simulink model "model"  (R2020a)
settings: Solver=VariableStepAuto  StartTime=0.0  StopTime=10  RelTol=1e-3
undefined symbols (not defined in the file): b, F, k1, k2, m1, m2
settings Model: Creator=PRATIKSHA  LastModifiedBy=PRATIKSHA

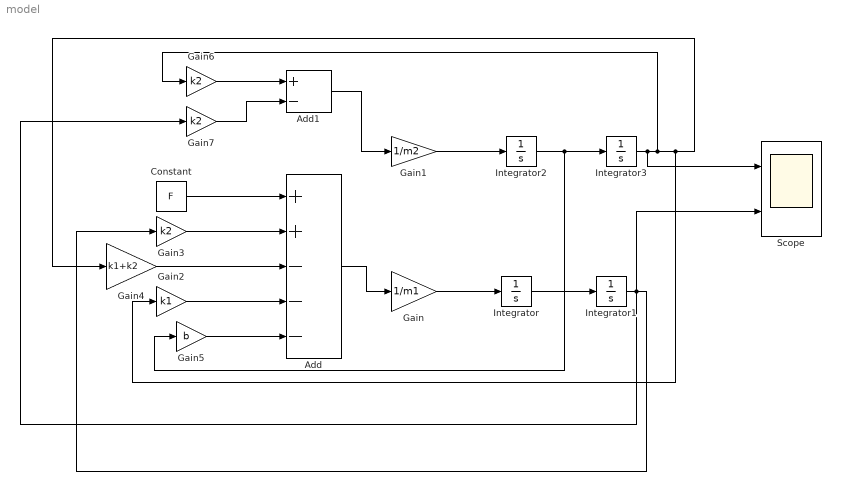
== system model ==
  Add : Sum  Inputs=++---
  Add1 : Sum  Inputs=+-
  Constant : Constant  Value=F
  Gain : Gain  Gain=1/m1
  Gain1 : Gain  Gain=1/m2
  Gain2 : Gain  Gain=k1
  Gain3 : Gain  Gain=k2
  Gain4 : Gain  Gain=k1+k2
  Gain5 : Gain  Gain=b
  Gain6 : Gain  Gain=k2
  Gain7 : Gain  Gain=k2
  Integrator{,1..3} (4 alike) : Integrator
  Scope : Scope  NumInputPorts=2
  wires:
  Constant/1 -> Add/1
  Gain/1 -> Integrator/1
  Integrator/1 -> Integrator1/1
  Add/1 -> Gain/1
  Gain2/1 -> Add/4
  Gain3/1 -> Add/2
  Gain4/1 -> Add/3
  Gain5/1 -> Add/5
  Integrator2/1 -> Gain5/1, Integrator3/1
  Gain1/1 -> Integrator2/1
  Gain6/1 -> Add1/1
  Gain7/1 -> Add1/2
  Integrator1/1 -> Scope/2, Gain7/1, Gain3/1
  Integrator3/1 -> Scope/1, Gain6/1, Gain2/1, Gain4/1
  Add1/1 -> Gain1/1
